simulink model "LAB3_fromLab2"  (R2020a)
settings: Solver=FixedStepDiscrete  StartTime=0.0  StopTime=60  FixedStep=0.05  RelTol=1e-3  EnableMultiTasking=on
settings Model: Creator=plavoie  LastModifiedBy=horia
settings DataIOCC: LimitDataPoints=on  SaveFormat=Array  SignalLoggingSaveFormat=ModelDataLogs  ReturnWorkspaceOutputs=off
settings OptimizationCC: ExpressionDepthLimit=2147483647  LifeSpan=inf
settings DebuggingCC: UnderspecifiedInitializationDetection=Classic  MergeDetectMultiDrivingBlocksExec=none  SolverPrmCheckMsg=warning  FcnCallInpInsideContextMsg=warning  StateNameClashWarn=warning  SFUnexpectedBacktrackingDiag=warning  SFNoUnconditionalDefaultTransitionDiag=warning  SFExecutionAtInitializationDiag=none  ArithmeticOperatorsInVariantConditions=warning
settings HardwareCC: ProdBitPerPointer=32  ProdBitPerSizeT=32  ProdBitPerPtrDiffT=32  ProdLargestAtomicFloat=None  ProdIntDivRoundTo=Undefined  ProdEndianess=Unspecified  ProdWordSize=32  ProdHWDeviceType=32-bit Generic
settings ModelReferenceCC: PropagateSignalLabelsOutOfModel=off
settings SFSimCC: SimUseLocalCustomCode=off  CustomCodeUndefinedFunction=UseInterfaceOnly
settings RTWCC: RTWUseLocalCustomCode=off
settings CodeAppCC: StateflowObjectComments=on
settings GRTTargetCC: TargetLangStandard=C89/C90 (ANSI)  CombineOutputUpdateFcns=off  GRTInterface=on
settings ConfigComp: CovMetricSettings=dw  CovHtmlReporting=on  CovSaveCumulativeToWorkspaceVar=on  CovSaveSingleToWorkspaceVar=on  CovExternalEMLEnable=off

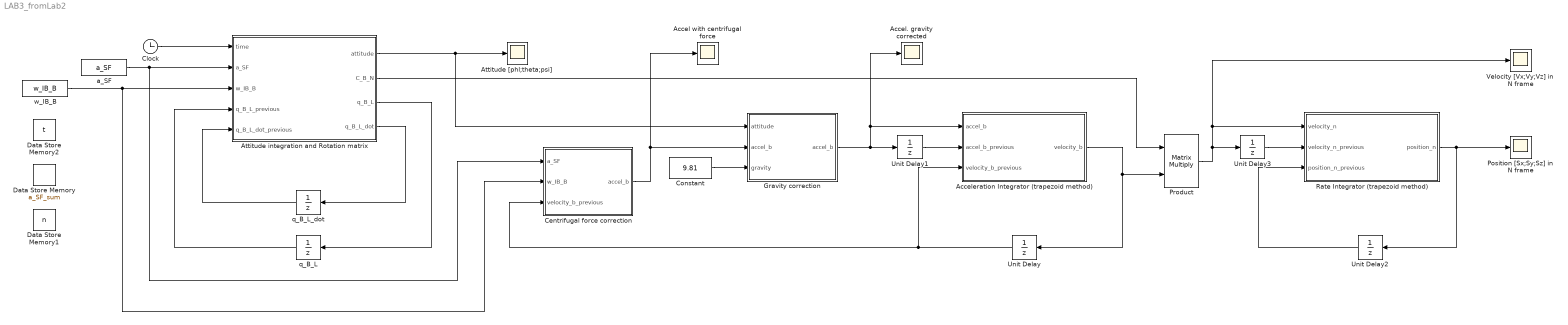
== system LAB3_fromLab2 ==
  Accel with centrifugal force : Scope
  Accel. gravity corrected : Scope
  Acceleration Integrator (trapezoid method) : MATLAB Function  TreatAsAtomicUnit=on
  Attitude [phl;theta;psi] : Scope
  Attitude integration and Rotation matrix : MATLAB Function  TreatAsAtomicUnit=on
  Centrifugal force correction : MATLAB Function  TreatAsAtomicUnit=on
  Clock : Clock
  Constant : Constant  Value=9.81
  Data Store Memory : DataStoreMemory  DataStoreName=a_SF_sum  ReadBeforeWriteMsg=warning  WriteAfterWriteMsg=warning  WriteAfterReadMsg=warning  ShowAdditionalParam=off  OutDataTypeStr=single  Dimensions=3
  Data Store Memory1 : DataStoreMemory  DataStoreName=n  ReadBeforeWriteMsg=warning  WriteAfterWriteMsg=warning  WriteAfterReadMsg=warning  ShowAdditionalParam=off  OutDataTypeStr=int8
  Data Store Memory2 : DataStoreMemory  DataStoreName=t  ReadBeforeWriteMsg=warning  WriteAfterWriteMsg=warning  WriteAfterReadMsg=warning  ShowAdditionalParam=off  OutDataTypeStr=single
  Gravity correction : MATLAB Function  TreatAsAtomicUnit=on
  Position [Sx;Sy;Sz] in N frame : Scope
  Product : Product  Multiplication=Matrix(*)
  Rate Integrator (trapezoid method) : MATLAB Function  TreatAsAtomicUnit=on
  Unit Delay{,1..3} (4 alike) : UnitDelay  InitialCondition=[0;0;0]  SampleTime=-1  HasFrameUpgradeWarning=on
  Velocity [Vx;Vy;Vz] in N frame : Scope
  a_SF : FromWorkspace  VariableName=a_SF
  q_B_L : UnitDelay  InitialCondition=[1;0;0;0]  SampleTime=-1  HasFrameUpgradeWarning=on
  q_B_L_dot : UnitDelay  InitialCondition=zeros(4,1)  SampleTime=-1  HasFrameUpgradeWarning=on
  w_IB_B : FromWorkspace  VariableName=w_IB_B
  wires:
  a_SF/1 -> Centrifugal force correction/1(a_SF), Attitude integration and Rotation matrix/2(a_SF)
  w_IB_B/1 -> Centrifugal force correction/2(w_IB_B), Attitude integration and Rotation matrix/3(w_IB_B)
  Clock/1 -> Attitude integration and Rotation matrix/1(time)
  Attitude integration and Rotation matrix/3(q_B_L) -> q_B_L/1
  q_B_L/1 -> Attitude integration and Rotation matrix/4(q_B_L_previous)
  Attitude integration and Rotation matrix/4(q_B_L_dot) -> q_B_L_dot/1
  q_B_L_dot/1 -> Attitude integration and Rotation matrix/5(q_B_L_dot_previous)
  Attitude integration and Rotation matrix/1(attitude) -> Attitude [phl;theta;psi]/1, Gravity correction/1(attitude)
  Constant/1 -> Gravity correction/3(gravity)
  Gravity correction/1(accel_b) -> Unit Delay1/1, Acceleration Integrator (trapezoid method)/1(accel_b), Accel. gravity corrected/1
  Centrifugal force correction/1(accel_b) -> Gravity correction/2("accel_b "), Accel with centrifugal force/1
  Product/1 -> Unit Delay3/1, Rate Integrator (trapezoid method)/1(velocity_n), Velocity [Vx;Vy;Vz] in N frame/1
  Acceleration Integrator (trapezoid method)/1(velocity_b) -> Product/2, Unit Delay/1
  Unit Delay/1 -> Centrifugal force correction/3(velocity_b_previous), Acceleration Integrator (trapezoid method)/3(velocity_b_previous)
  Unit Delay1/1 -> Acceleration Integrator (trapezoid method)/2(accel_b_previous)
  Attitude integration and Rotation matrix/2(C_B_N) -> Product/1
  Rate Integrator (trapezoid method)/1(position_n) -> Unit Delay2/1, Position [Sx;Sy;Sz] in N frame/1
  Unit Delay2/1 -> Rate Integrator (trapezoid method)/3(position_n_previous)
  Unit Delay3/1 -> Rate Integrator (trapezoid method)/2(velocity_n_previous)

== matlab function LAB3_fromLab2/Attitude integration and Rotation matrix ==
  data: time input; a_SF input; attitude output; w_IB_B input; C_B_N output; q_B_L_previous input; q_B_L_dot_previous input; q_B_L output; q_B_L_dot output
function [attitude,C_B_N,q_B_L,q_B_L_dot] = fcn(time,a_SF,w_IB_B,q_B_L_previous,q_B_L_dot_previous)
%phi,theta,psi
%-- Partie initialisation ---------------------
persistent FlagInit counteur
attitude = [0;0;0];
q_B_L = q_B_L_previous ;
q_B_L_dot = q_B_L_dot_previous  ;
a_SF_sum = zeros(1,3);
C_B_N = zeros(3,3);

%%%%%%%%%%%%%%%%%%%%%%%%%%%%%%%%%%%%%%%%%%%%%%%%%%%%%%%%%%%%%%%%%%%%%%%%%%%
%
%  function R=q2dcm(q)
%
%>
%> @brief Function that converts a  quaternion vector to a directional
%> cosine matrix (rotation matrix) 
%>
%> @param[out]   R      Rotation matrix.
%> @param[in]    q      Quaternion vector.
%>
%
%%%%%%%%%%%%%%%%%%%%%%%%%%%%%%%%%%%%%%%%%%%%%%%%%%%%%%%%%%%%%%%%%%%%%%%%%%%
function R=q2dcm(q)

R = zeros(3,3);
p=zeros(6,1);

p(1:4)=q.^2;

p(5)=p(2)+p(3);

if p(1)+p(4)+p(5)~=0
   p(6)=2/(p(1)+p(4)+p(5)); 
else
   p(6)=0;
end


R(1,1)=1-p(6)*p(5);
R(2,2)=1-p(6)*(p(1)+p(3));
R(3,3)=1-p(6)*(p(1)+p(2));

p(1)=p(6)*q(1); 
p(2)=p(6)*q(2);
p(5)=p(6)*q(3)*q(4);
p(6)=p(1)*q(2);

R(1,2)=p(6)-p(5);
R(2,1)=p(6)+p(5);

p(5)=p(2)*q(4);
p(6)=p(1)*q(3);

R(1,3)=p(6)+p(5);
R(3,1)=p(6)-p(5);

p(5)=p(1)*q(4);
p(6)=p(2)*q(3);

R(2,3)=p(6)-p(5);
R(3,2)=p(6)+p(5);

end

%%%%%%%%%%%%%%%%%%%%%%%%%%%%%%%%%%%%%%%%%%%%%%%%%%%%%%%%%%%%%%%%%%%%%%%%%%%
%
%  function q=dcm2q(R)
%
%>
%> @brief Function that converts a directional cosine matrix (rotation 
%> matrix) in to a quaternion vector. 
%>
%> @param[out]    q      Quaternion vector.
%> @param[in]   R      Rotation matrix.
%>
%
%%%%%%%%%%%%%%%%%%%%%%%%%%%%%%%%%%%%%%%%%%%%%%%%%%%%%%%%%%%%%%%%%%%%%%%%%%%
function q=dcm2q(R)

T = 1 + R(1,1) + R(2,2) + R(3,3);

if T > 10^-8
    
    S = 0.5 / sqrt(T);
    qw = 0.25 / S;
    qx = ( R(3,2) - R(2,3) ) * S;
    qy = ( R(1,3) - R(3,1) ) * S;
    qz = ( R(2,1) - R(1,2) ) * S;

else
    
    if (R(1,1) > R(2,2)) && (R(1,1) > R(3,3))
        
        S = sqrt( 1 + R(1,1) - R(2,2) - R(3,3)) * 2; % S=4*qx
        qw = (R(3,2) - R(2,3)) / S;
        qx = 0.25 * S;
        qy = (R(1,2) + R(2,1)) / S;
        qz = (R(1,3) + R(3,1)) / S;
        
    elseif (R(2,2) > R(3,3))
        
        S = sqrt( 1 + R(2,2) - R(1,1) - R(3,3) ) * 2; %S=4*qy
        qw = (R(1,3) - R(3,1)) / S;
        qx = (R(1,2) + R(2,1)) / S;
        qy = 0.25 * S;
        qz = (R(2,3) + R(3,2)) / S;

    else
        
        S = sqrt( 1 + R(3,3) - R(1,1) - R(2,2) ) * 2; % S=4*qz
        qw = (R(2,1) - R(1,2)) / S;
        qx = (R(1,3) + R(3,1)) / S;
        qy = (R(2,3) + R(3,2)) / S;
        qz = 0.25 * S;

    end

end

%Store in vector
q = [qx qy qz qw]';
end



%-------------- La magnitude de l'acceleration est definie par :-----
acc_mag = sqrt(a_SF(1)^2 + a_SF(2)^2 + a_SF(3)^2);
%----------Par définition, l’axe Z du repère L est orienté selon gP
AxeZ_SF = - a_SF / acc_mag; 

%--------Init Matrix------------------
if isempty(FlagInit) && isempty(counteur)
%-- Initialisation des composentes Euler et la marice DCM
    a_SF_sum(1) =  AxeZ_SF(1);
    a_SF_sum(2) =  AxeZ_SF(2);
    a_SF_sum(3) =  AxeZ_SF(3);
%     for i = 1:3
%         a_SF_sum(i) = 0;
%     end
    FlagInit = 0;
    counteur = 0;
end

%En supposant que le système est stationnaire pendant les 25 premiers
%échantillons, le roulis et le tangage initiaux sont calculés à partir 
%des 25 premiers lectures de l'accéléromètre.
% Determination de l'Alttitude 
if (FlagInit == 0)
C_B_L = zeros(3);
%---- Initialisation par Alignement Grossier------
    C_B_L(3,1) = a_SF_sum(1);
    C_B_L(3,2) = a_SF_sum(2);
    C_B_L(3,3) = a_SF_sum(3);
    K = 1/sqrt(C_B_L(3,2)^2+C_B_L(3,3)^2);
    C_B_L(2,1) = 0;
    C_B_L(2,2) = K * C_B_L(3,3);
    C_B_L(2,3) =-K * C_B_L(3,2);
    C_B_L(1,1) = C_B_L(2,2) * C_B_L(3,3) - C_B_L(2,3) * C_B_L(3,2);
    C_B_L(1,2) = C_B_L(2,3) * C_B_L(3,1) - C_B_L(2,1) * C_B_L(3,3);
    C_B_L(1,3) = C_B_L(2,1) * C_B_L(3,2) - C_B_L(2,2) * C_B_L(3,1);
    C_B_L = [C_B_L(1,1) C_B_L(1,2) C_B_L(1,3); C_B_L(2,1) C_B_L(2,2) C_B_L(2,3); C_B_L(3,1) C_B_L(3,2) C_B_L(3,3)];
    %calculate initial quaternion from C_B_L matrix
    C_B_N = C_B_L;
    q_B_L = dcm2q(C_B_L);
    %calculate euler angles phi, theta, psi
    psi = atan2( 2 *( q_B_L(2) * q_B_L(3) - q_B_L(1) * q_B_L(4)) , 2 * (q_B_L(1)^2 + q_B_L(1)^2) - 1 ) * 180/pi ;
    theta = - asin( 2 *(q_B_L(2) * q_B_L(4) + q_B_L(1) * q_B_L(3))) * 180/pi;
    phi = atan2( 2* (q_B_L(3) * q_B_L(4) - q_B_L(1) * q_B_L(2)) , 2 * (q_B_L(1)^2 + q_B_L(4)^2) - 1 ) * 180/pi;
    attitude = [phi;theta;psi];
    FlagInit = 1;
elseif FlagInit == 1
%Create skew symetric matrix of gyroscope output
   Qw_B_IB_Mat =[    0       -w_IB_B(1)    -w_IB_B(2)    -w_IB_B(3);
             w_IB_B(1)       0         -w_IB_B(3)     w_IB_B(2);
             w_IB_B(2)   w_IB_B(3)         0         -w_IB_B(1);
             w_IB_B(3)  -w_IB_B(2)     w_IB_B(1)          0    ];

    q_L_B = transpose([q_B_L(1) ;q_B_L(2); q_B_L(3); q_B_L(4)]);
%Variation du quaternion
    q_B_L_dot = 0.5 * Qw_B_IB_Mat * q_B_L;
            
    q_B_L_dot = [ q_B_L_dot(1); q_B_L_dot(2); q_B_L_dot(3); q_B_L_dot(4)];
%trapezoidal integration to get new q_B_L 
%---- Équations de propagation d'attitude             
%---- Trapezoide integre q_B_L
    q_B_L = q_B_L_previous + (0.01/2) *( q_B_L_dot + q_B_L_dot_previous );
    C_B_N = q2dcm(q_B_L);
%Calcule de la variation d'Attitude Quaternion 
    psi = atan2( 2 *( q_B_L(2) * q_B_L(3) - q_B_L(1) * q_B_L(4)) , 2 * (q_B_L(1)^2 + q_B_L(2)^2) - 1 ) * 180/pi ;
    theta = - asin( 2 *(q_B_L(2) * q_B_L(4) + q_B_L(1) * q_B_L(3))) * 180/pi;
    phi = atan2( 2* (q_B_L(3) * q_B_L(4) - q_B_L(1) * q_B_L(2)) , 2 * (q_B_L(1)^2 + q_B_L(4)^2) - 1 ) * 180/pi;
    
    attitude = [phi;theta;psi];
    
end

end

== matlab function LAB3_fromLab2/Acceleration Integrator (trapezoid method) ==
  data: accel_b input; velocity_b output; accel_b_previous input; velocity_b_previous input
function velocity_b=fcn(accel_b,accel_b_previous,velocity_b_previous)
                            
velocity_b = velocity_b_previous + (0.01/2) * (accel_b + accel_b_previous);

end

== matlab function LAB3_fromLab2/Centrifugal force correction ==
  data: a_SF input; w_IB_B input; velocity_b_previous input; accel_b output
function accel_b=fcn(a_SF,w_IB_B,velocity_b_previous)

accel_b_x = a_SF(1) - w_IB_B(1) * velocity_b_previous(1);
accel_b_y = a_SF(2) - w_IB_B(2) * velocity_b_previous(2);
accel_b_z = a_SF(3) - w_IB_B(3) * velocity_b_previous(3);

accel_b = [accel_b_x;accel_b_y;accel_b_z];

end

== matlab function LAB3_fromLab2/Gravity correction ==
  data: attitude input; accel_b input; gravity input; accel_b output
function accel_b=fcn(attitude,accel_b,gravity)
                            
accel_b_x = accel_b(1) + gravity * -sin(attitude(2)*pi/180);
accel_b_y = accel_b(2) + gravity * cos(attitude(2)*pi/180) * sin(attitude(1)*pi/180);
accel_b_z = accel_b(3) + gravity * cos(attitude(2)*pi/180) * cos(attitude(1)*pi/180);

accel_b = [accel_b_x;accel_b_y;accel_b_z];

end

== matlab function LAB3_fromLab2/Rate Integrator (trapezoid method) ==
  data: velocity_n input; position_n output; velocity_n_previous input; position_n_previous input
function position_n=fcn(velocity_n,velocity_n_previous,position_n_previous)
                            
position_n = position_n_previous + (0.01/2) * (velocity_n + velocity_n_previous);

end
